simulink model "acdcmg_sim8_1_sm_grid_simulation"  (R2019b)
settings: Solver=ode8  StartTime=0.0  StopTime=0.5  FixedStep=4e-05  MaxStep=1e-2  RelTol=1e-3
PreLoadFcn:
  | Set_parameters_R2018
InitFcn:
  | Set_parameters_R2018
undefined symbols (not defined in the file or in its folder): D1, Delta, dis11, dis12, dis2, dis3, dis4, dis5, dis6, DiscIntNeverNeededParam, fn, Fnom, Ion, Lithium, max_min, P_Load_3, Pnom_T1, Pnom_T2, Pnom_T3, Ql_Load_3, R_Load_9, R_Load_DC, Rl, Rls, Ts, Ts_Control, Ts_Power, Ts_PV, V1_LL_T3, Vmin_mppt, VnInv, Vnom_DC, Vnom_Diesel, Vnom_prim, Vnom_sec, Vnom_ter_AC_DC, Xl, Xls
libraries: powerlib x136, powerlib_meascontrol x67, opal_lib x24, artemis x7, simulink x7, powerlib_extras x5, electricdrivelib x1, eeSinusoidalMeasurementV2 x1, re_lib x1
(part 4 of 4)

== system acdcmg_sim8_1_sm_grid_simulation/SM_Grid_Simulation/Bus_AC//DC3/Battery system/Ripple Calculations ==
  Signal : Inport
  Reset : Inport  Port=2
  0 : Constant  Value=2
  1 : Constant  Value=2
  Display10 : Display
  Display2 : Display
  Mean1 : powerlib_meascontrol/Measurements/Mean  Freq=10  Vinit=0  Ts=0
  MinMax Running Resettable : simulink/Math Operations/MinMax Running Resettable  Function=max  vinit=0.0
  MinMax Running Resettable1 : simulink/Math Operations/MinMax Running Resettable  Function=min  vinit=0.0
  Product : Product
  Product1 : Product
  Sum : Sum  Inputs=|+-
  Sum1 : Sum  Inputs=|-+
  Switch1 : Switch  Criteria=u2 > Threshold
  Switch2 : Switch  Criteria=u2 > Threshold
  Switch3 : Switch  Criteria=u2 > Threshold
  Ripple in Buck : Outport  VectorParamsAs1DForOutWhenUnconnected=off
  Ripple in Boost : Outport  Port=2  VectorParamsAs1DForOutWhenUnconnected=off
  wires:
  1/1 -> Product1/2
  [I_ref] -> Switch2/2, Switch3/2
  Product1/1 -> Switch3/3
  0/1 -> Product/2
  Switch2/1 -> Ripple in Buck/1
  Switch3/1 -> Ripple in Boost/1
  Product/1 -> Switch2/1
  Signal/1 -> Mean1/1, MinMax Running Resettable1/1, MinMax Running Resettable/1
  Switch1/1 -> Sum1/2, Sum/2
  MinMax Running Resettable/1 -> Sum/1, Display2/1
  MinMax Running Resettable1/1 -> Sum1/1, Display10/1
  Sum/1 -> Product/1
  Reset/1 -> Switch1/2, MinMax Running Resettable1/2, MinMax Running Resettable/2
  Sum1/1 -> Product1/1
  Mean1/1 -> Switch1/3

== system acdcmg_sim8_1_sm_grid_simulation/SM_Grid_Simulation/Bus_AC//DC3/PV system/Pmean ==
  Product : Product  RndMeth=Zero
  Scope : Scope  NumInputPorts=2
  W-kW : Gain  Gain=1/1000
  P : Outport  VectorParamsAs1DForOutWhenUnconnected=off
  V : Outport  Port=2  VectorParamsAs1DForOutWhenUnconnected=off
  wires:
  [Vdc_PV] -> Scope/1, Product/1, V/1
  Product/1 -> W-kW/1
  [Idc_PV] -> Scope/2, Product/2
  W-kW/1 -> P/1  "Pmean_PV (kW)"

== system acdcmg_sim8_1_sm_grid_simulation/SM_Grid_Simulation/Grid Bi-directional Converter 1.1 300 (DC) // 150 V (AC) P_nom 3kW2/Control of Inverter/Discrete PWM Generator1 ==
  note: Pierre Giroux, Gilbert Sybille
      | Power System Laboratory, IREQ
      | Hydro-Quebec
  note: PWM Generator
  Uref : Inport
  BL4 : Logic  Operator=NOT  Inputs=1
  BL5 : Logic  Operator=NOT  Inputs=1
  Constant : Constant  Value=Internal_Phase
  Constant1 : Constant  Value=Internal
  Data Type Conversion : DataTypeConversion  OutDataTypeStr=double  SaturateOnIntegerOverflow=on  RndMeth=Zero
  Data Type Conversion1 : DataTypeConversion  OutDataTypeStr=boolean  SaturateOnIntegerOverflow=on  RndMeth=Zero
  Data Type Conversion2 : DataTypeConversion  OutDataTypeStr=boolean  SaturateOnIntegerOverflow=on  RndMeth=Zero
  Gain : Gain  Gain=2*pi*Freq  SaturateOnIntegerOverflow=on  OutDataTypeStr=Inherit: Same as input  ParamDataTypeStr=Inherit: Same as input
  Gain2 : Gain  Gain=pi/180  SaturateOnIntegerOverflow=on  OutDataTypeStr=Inherit: Same as input  ParamDataTypeStr=Inherit: Same as input
  Gain3 : Gain  Gain=-1  SaturateOnIntegerOverflow=on  OutDataTypeStr=Inherit: Same as input  ParamDataTypeStr=Inherit: Same as input
  Mux : Mux  Inputs=2
  Mux1 : Mux  Inputs=2
  Mux2 : Mux  Inputs=2
  Product : Product  SaturateOnIntegerOverflow=on  InputSameDT=on  OutDataTypeStr=Inherit: Same as first input
  Relational Operator : RelationalOperator  RndMeth=Nearest  InputSameDT=on
  Relational Operator1 : RelationalOperator  RndMeth=Nearest  InputSameDT=on
  Select1A : Selector  InputPortWidth=Select1_PortWidth  IndexOptions=Index vector (dialog)  Indices=Select1_Elements  OutputSizes=1
  Select1B : Selector  InputPortWidth=Select1_PortWidth  IndexOptions=Index vector (dialog)  Indices=Select1_Elements  OutputSizes=1
  Select3 : Selector  InputPortWidth=Select3_PortWidth  IndexOptions=Index vector (dialog)  Indices=Select3_Elements  OutputSizes=1
  Sum : Sum  Inputs=+++  SaturateOnIntegerOverflow=on  InputSameDT=on  OutDataTypeStr=Inherit: Same as first input
  Switch : Switch  Criteria=u2 > Threshold
  Triangle : simulink/Sources/Repeating Sequence  rep_seq_t=[0 1/Fc/4 3/Fc/4 1/Fc]  rep_seq_y=[0 -1 1 0]
  Trigonometric Function : Trigonometry
  m3 : Constant  Value=Phase
  m4 : Constant  Value=mIndex
  t : DigitalClock  SampleTime=Ts
  Pulses : Outport  VectorParamsAs1DForOutWhenUnconnected=off
  wires:
  Mux2/1 -> Select3/1
  Select1B/1 -> Mux2/2
  Select1A/1 -> Mux2/1
  Mux1/1 -> Select1B/1
  Mux/1 -> Select1A/1
  BL5/1 -> Mux1/2
  BL4/1 -> Mux/2
  Gain3/1 -> Relational Operator1/1
  Triangle/1 -> Relational Operator1/2, Relational Operator/2
  Product/1 -> Switch/1
  Constant1/1 -> Switch/2
  Trigonometric Function/1 -> Product/2
  Sum/1 -> Trigonometric Function/1
  m4/1 -> Product/1
  Constant/1 -> Sum/3
  m3/1 -> Gain2/1
  Gain2/1 -> Sum/2
  Gain/1 -> Sum/1
  t/1 -> Gain/1
  Select3/1 -> Data Type Conversion/1
  Data Type Conversion/1 -> Pulses/1
  Relational Operator/1 -> Data Type Conversion1/1
  Data Type Conversion1/1 -> BL4/1, Mux/1
  Relational Operator1/1 -> Data Type Conversion2/1
  Data Type Conversion2/1 -> BL5/1, Mux1/1
  Switch/1 -> Relational Operator/1, Gain3/1
  Uref/1 -> Switch/3

== system acdcmg_sim8_1_sm_grid_simulation/SM_Grid_Simulation/Grid Bi-directional Converter 1.1 300 (DC) // 150 V (AC) P_nom 3kW2/Control of Inverter/MI Controller ==
  Vabc : Inport
  Demux : Demux  Commented=on  Outputs=3
  Demux1 : Demux  Outputs=3
  Mux : Mux  Inputs=3
  Mux1 : Mux  Inputs=3
  Mux2 : Mux  Inputs=3
  OP max / min : Subsystem
  Product : Product  RndMeth=Zero
  Product1 : Product  RndMeth=Zero
  Product2 : Product  RndMeth=Zero
  Subsystem : Subsystem
  Subsystem1 : Subsystem
  Terminator : Terminator
  Terminator1 : Terminator  Commented=on
  Terminator2 : Terminator  Commented=on
  Terminator3 : Terminator
  Terminator4 : Terminator  Commented=on
  Vab1 : powerlib_extras/Discrete Measurements/Discrete  RMS value  Commented=on  Freq=60  Mag_Init=0  Ts=20e-6
      settings: SourceProductBaseCode=PS
  Vab5 : powerlib_extras/Discrete Measurements/Discrete  RMS value  Commented=on  Freq=60  Mag_Init=0  Ts=20e-6
      settings: SourceProductBaseCode=PS
  Vab6 : powerlib_extras/Discrete Measurements/Discrete  RMS value  Commented=on  Freq=60  Mag_Init=0  Ts=20e-6
      settings: SourceProductBaseCode=PS
  Vabc_inv : Outport  VectorParamsAs1DForOutWhenUnconnected=off
  u / m : Outport  Port=2  VectorParamsAs1DForOutWhenUnconnected=off
  wires:
  Product/1 -> Mux2/1
  Product1/1 -> Mux2/2
  Product2/1 -> Mux2/3
  Mux1/1 -> u / m/1
  Vabc/1 -> Demux/1
  Demux/1 -> Vab6/1
  Demux/2 -> Vab5/1
  Demux/3 -> Vab1/1
  Demux1/1 -> Product/1, Mux1/1
  Demux1/2 -> Product1/1, Mux1/2
  Demux1/3 -> Product2/1, Mux1/3
  Subsystem/1(Va) -> Product/2
  Subsystem/2(Vb) -> Product1/2
  Subsystem/3(Vc) -> Product2/2
  Mux2/1 -> Vabc_inv/1
  Vab6/1 -> Terminator2/1
  Subsystem1/3(wt) -> Terminator/1
  Subsystem1/1(Frec) -> Terminator3/1
  Subsystem1/2(sin_cos) -> Subsystem/1(sin_cos)
  Mux/1 -> Demux1/1
  OP max / min/1(ctrl) -> Mux/3, Mux/1, Mux/2
  Vab5/1 -> Terminator1/1
  Vab1/1 -> Terminator4/1

== system acdcmg_sim8_1_sm_grid_simulation/SM_Grid_Simulation/Inverter 300 (DC) // 150 V (AC) P_nom 10 kW4/Control of Inverter/Positive-Sequence Active & Reactive Power1 ==
  note: Discrete 3-phase Positive-Sequence Active & Reactive Power
  note: Pierre Giroux, Gilbert Sybille
      | Power System Simulation Laboratory
      | IREQ, Hydro-Quebc
  Vabc : Inport  PortDimensions=3
  Iabc : Inport  Port=2  PortDimensions=3
  Deg->Rad : Gain  Gain=pi/180  SaturateOnIntegerOverflow=on  OutDataTypeStr=Inherit: Same as input  ParamDataTypeStr=Inherit: Same as input
  Discrete 3-phase Positive-Sequence Fundamental Value (I) : powerlib_extras/Discrete Measurements/Discrete 3-phase Positive-Sequence Fundamental Value  Freq=Freq  Par_Init=Par_Iinit  Ts=Ts
      settings: SourceProductBaseCode=PS
  Discrete 3-phase Positive-Sequence Fundamental Value (V) : powerlib_extras/Discrete Measurements/Discrete 3-phase Positive-Sequence Fundamental Value  Freq=Freq  Par_Init=Par_Vinit  Ts=Ts
      settings: SourceProductBaseCode=PS
  Gain1 : Gain  Gain=3/2  SaturateOnIntegerOverflow=on  OutDataTypeStr=Inherit: Same as input  ParamDataTypeStr=Inherit: Same as input
  Mag->RMS : Gain  Gain=1/sqrt(2)
  Mux1 : Mux  Inputs=2
  Mux2 : Mux  Inputs=2
  Mux3 : Mux  Inputs=2
  Product : Product  SaturateOnIntegerOverflow=on  InputSameDT=on  OutDataTypeStr=Inherit: Same as first input
  Product1 : Product  SaturateOnIntegerOverflow=on  InputSameDT=on  OutDataTypeStr=Inherit: Same as first input
  Product2 : Product  SaturateOnIntegerOverflow=on  InputSameDT=on  OutDataTypeStr=Inherit: Same as first input
  Sum : Sum  Inputs=+-  SaturateOnIntegerOverflow=on  InputSameDT=on  OutDataTypeStr=Inherit: Same as first input
  Trigonometric Function : Trigonometry
  Trigonometric Function1 : Trigonometry  Operator=cos
  W->kW Var->kvar : Gain  Gain=1/1000
  RMS_V_I : Outport
  P_Q(kW) : Outport  Port=2
  Phase_V_I : Outport  Port=3
  PF : Outport  Port=4
  wires:
  Vabc/1 -> Discrete 3-phase Positive-Sequence Fundamental Value (V)/1
  Iabc/1 -> Discrete 3-phase Positive-Sequence Fundamental Value (I)/1
  Discrete 3-phase Positive-Sequence Fundamental Value (V)/2 -> Sum/1, Mux1/1
  Discrete 3-phase Positive-Sequence Fundamental Value (I)/2 -> Sum/2, Mux1/2
  Sum/1 -> Deg->Rad/1
  Deg->Rad/1 -> Trigonometric Function1/1, Trigonometric Function/1
  Trigonometric Function1/1 -> PF/1, Product/2
  Trigonometric Function/1 -> Product1/1
  Mux2/1 -> Gain1/1
  Product/1 -> Mux2/1
  Product1/1 -> Mux2/2
  Product2/1 -> Product/1, Product1/2
  Discrete 3-phase Positive-Sequence Fundamental Value (V)/1 -> Mux3/1, Product2/1
  Discrete 3-phase Positive-Sequence Fundamental Value (I)/1 -> Mux3/2, Product2/2
  Mux1/1 -> Phase_V_I/1
  Mux3/1 -> Mag->RMS/1
  Mag->RMS/1 -> RMS_V_I/1
  Gain1/1 -> W->kW Var->kvar/1
  W->kW Var->kvar/1 -> P_Q(kW)/1

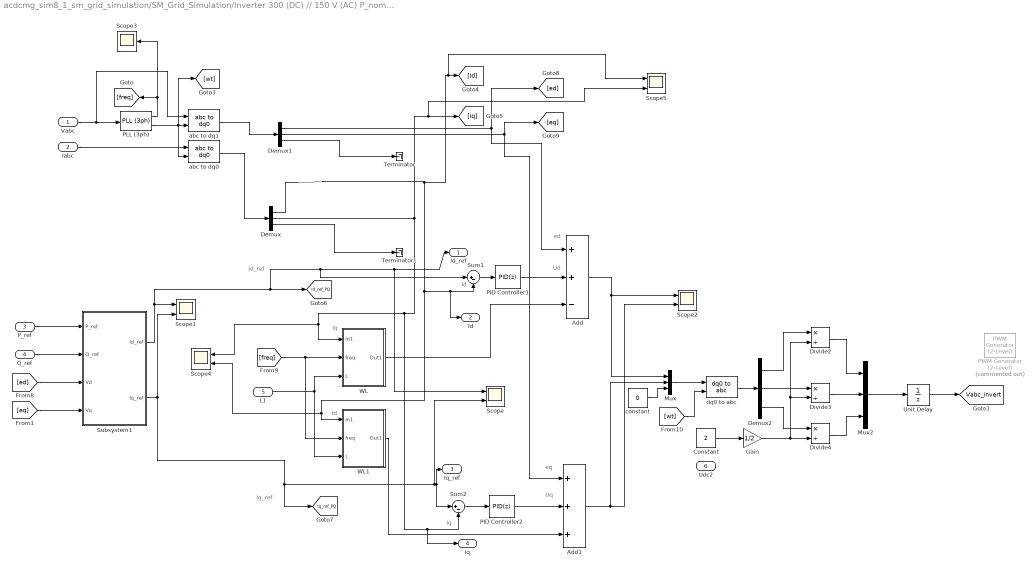
== system acdcmg_sim8_1_sm_grid_simulation/SM_Grid_Simulation/Inverter 300 (DC) // 150 V (AC) P_nom 10 kW4/Control of Inverter/Subsystem2 ==
  note: Iq_ref
  note: Id
  note: Id_ref
  note: Ud
  note: Uq
  note: eq
  note: ed
  note: Iq
  note: Id
  note: Iq
  Vabc : Inport
  Iabc : Inport  Port=2
  P_ref : Inport  Port=3
  Q_ref : Inport  Port=4
  L1 : Inport  Port=5
  Udc2 : Inport  Port=6
  Add : Sum  Inputs=++-
  Add1 : Sum  Inputs=+++
  Constant : Constant  Value=2
  Demux : Demux  Outputs=3
  Demux1 : Demux  Outputs=3
  Demux2 : Demux  Outputs=3
  Divide2 : Product  Inputs=*/
  Divide3 : Product  Inputs=*/
  Divide4 : Product  Inputs=*/
  Gain : Gain  Gain=1/2
  Mux : Mux  Inputs=3
  Mux2 : Mux  Inputs=3
  PID Controller1 : simulink/Continuous/PID Controller  Controller=PID  Form=Parallel  TimeDomain=Discrete-time  SampleTime=Ts_Control  IntegratorMethod=Forward Euler  FilterMethod=Forward Euler  ControllerParametersSource=internal  P=Kp  I=Ki  D=Kd  UseFilter=on  N=100  TunerSelectOption=Transfer Function Based (PID Tuner App)  InitialConditionSource=internal  InitialConditionForIntegrator=0  InitialConditionForFilter=0  DifferentiatorICPrevScaledInput=0  ExternalReset=none  TrackingMode=off  Kt=1  LimitOutput=off  UpperSaturationLimit=inf  LowerSaturationLimit=-inf  LinearizeAsGain=on  AntiWindupMode=none  Kb=1  POutMin=[]  POutMax=[]  IOutMin=[]  IOutMax=[]  DOutMin=[]  DOutMax=[]  NOutMin=[]  NOutMax=[]  SumOutMin=[]  SumOutMax=[]  SaturationOutMin=[]  SaturationOutMax=[]  PParamMin=[]  PParamMax=[]  IParamMin=[]  IParamMax=[]  DParamMin=[]  DParamMax=[]  NParamMin=[]  NParamMax=[]  KbParamMin=[]  KbParamMax=[]  KtParamMin=[]  KtParamMax=[]  KbOutMin=[]  KbOutMax=[]  KtOutMin=[]  KtOutMax=[]  IntegratorOutMin=[]  IntegratorOutMax=[]  FilterOutMin=[]  FilterOutMax=[]  SumI1OutMin=[]  SumI1OutMax=[]  SumI2OutMin=[]  SumI2OutMax=[]  SumI3OutMin=[]  SumI3OutMax=[]  SumI4OutMin=[]  SumI4OutMax=[]  SumDOutMin=[]  SumDOutMax=[]  DifferentiatorOutMin=[]  DifferentiatorOutMax=[]  FilterDiffOutCoefMin=[]  FilterDiffOutCoefMax=[]  ReciprocalOutMin=[]  ReciprocalOutMax=[]  SumDenOutMin=[]  SumDenOutMax=[]  SumNumOutMin=[]  SumNumOutMax=[]  DivideOutMin=[]  DivideOutMax=[]  IntegratorContinuousStateAttributes=''  IntegratorStateMustResolveToSignalObject=off  IntegratorRTWStateStorageClass=Auto  FilterContinuousStateAttributes=''  FilterStateMustResolveToSignalObject=off  FilterRTWStateStorageClass=Auto  ParallelPVariant=InternalParameters  IdealPVariant=Disabled  IVariant=InternalParameters  DVariant=InternalParameters  IntegratorVariant=Discrete  SatVariant=Disabled  AWVariant=Passthrough  PCopyVariant=Disabled  TRVariant=Disabled  FdbkBlocksVariant=Forward  IdealPFdbkVariant=Disabled  SatFdbkVariant=Disabled  DerivativeFilterVariant=ForwardEulerFilter  NVariant=InternalParameters  NCopyVariant=Disabled  FilterICVariant=InternalICsFilter  IntegratorICVariant=InternalICs  ExternalResetVariant=Disabled  TRSumVariant=Passthrough  SumFdbkVariant=Disabled  SumVariant=Sum_PID
  PID Controller2 : simulink/Continuous/PID Controller  Controller=PID  Form=Parallel  TimeDomain=Discrete-time  SampleTime=Ts_Control  IntegratorMethod=Forward Euler  FilterMethod=Forward Euler  ControllerParametersSource=internal  P=Kp  I=Ki  D=Kd  UseFilter=on  N=100  TunerSelectOption=Transfer Function Based (PID Tuner App)  InitialConditionSource=internal  InitialConditionForIntegrator=0  InitialConditionForFilter=0  DifferentiatorICPrevScaledInput=0  ExternalReset=none  TrackingMode=off  Kt=1  LimitOutput=off  UpperSaturationLimit=inf  LowerSaturationLimit=-inf  LinearizeAsGain=on  AntiWindupMode=none  Kb=1  POutMin=[]  POutMax=[]  IOutMin=[]  IOutMax=[]  DOutMin=[]  DOutMax=[]  NOutMin=[]  NOutMax=[]  SumOutMin=[]  SumOutMax=[]  SaturationOutMin=[]  SaturationOutMax=[]  PParamMin=[]  PParamMax=[]  IParamMin=[]  IParamMax=[]  DParamMin=[]  DParamMax=[]  NParamMin=[]  NParamMax=[]  KbParamMin=[]  KbParamMax=[]  KtParamMin=[]  KtParamMax=[]  KbOutMin=[]  KbOutMax=[]  KtOutMin=[]  KtOutMax=[]  IntegratorOutMin=[]  IntegratorOutMax=[]  FilterOutMin=[]  FilterOutMax=[]  SumI1OutMin=[]  SumI1OutMax=[]  SumI2OutMin=[]  SumI2OutMax=[]  SumI3OutMin=[]  SumI3OutMax=[]  SumI4OutMin=[]  SumI4OutMax=[]  SumDOutMin=[]  SumDOutMax=[]  DifferentiatorOutMin=[]  DifferentiatorOutMax=[]  FilterDiffOutCoefMin=[]  FilterDiffOutCoefMax=[]  ReciprocalOutMin=[]  ReciprocalOutMax=[]  SumDenOutMin=[]  SumDenOutMax=[]  SumNumOutMin=[]  SumNumOutMax=[]  DivideOutMin=[]  DivideOutMax=[]  IntegratorContinuousStateAttributes=''  IntegratorStateMustResolveToSignalObject=off  IntegratorRTWStateStorageClass=Auto  FilterContinuousStateAttributes=''  FilterStateMustResolveToSignalObject=off  FilterRTWStateStorageClass=Auto  ParallelPVariant=InternalParameters  IdealPVariant=Disabled  IVariant=InternalParameters  DVariant=InternalParameters  IntegratorVariant=Discrete  SatVariant=Disabled  AWVariant=Passthrough  PCopyVariant=Disabled  TRVariant=Disabled  FdbkBlocksVariant=Forward  IdealPFdbkVariant=Disabled  SatFdbkVariant=Disabled  DerivativeFilterVariant=ForwardEulerFilter  NVariant=InternalParameters  NCopyVariant=Disabled  FilterICVariant=InternalICsFilter  IntegratorICVariant=InternalICs  ExternalResetVariant=Disabled  TRSumVariant=Passthrough  SumFdbkVariant=Disabled  SumVariant=Sum_PID
  PLL (3ph) : powerlib_meascontrol/PLL/PLL (3ph)  Fmin=59.5  Par_Init=[0, 60]  ParK=[180, 3200, 1]  TcD=2.5e-4  MaxRateChangeFreq=12  FilterCutOffFreq=25  Ts=Ts_Control  AGC=on
  PWM Generator (2-Level) : powerlib_meascontrol/Pulse & Signal Generators/PWM Generator (2-Level)  Commented=on  ModulatorType=Three-phase bridge (6 pulses)  ModulatorMode=Unsynchronized  Fc=15000  Pc=90  nF=27  MinMax="[ -1  1 ]"  SamplingTechnique=Natural  ModulatingSignals=off  m=0.8  Freq=60  Phase=0  Ts=Ts_Power  ShowCarrierOutport=off
  Scope{,1..2,4..5} (5 alike) : Scope  NumInputPorts=2
  Scope3 : Scope
  Subsystem1 : Subsystem
  Sum1 : Sum  Inputs=|+-
  Sum2 : Sum  Inputs=|+-
  Terminator : Terminator
  Terminator1 : Terminator
  Unit Delay : UnitDelay  SampleTime=-1  HasFrameUpgradeWarning=on
  WL : Subsystem
  WL1 : Subsystem
  abc to dq0 : powerlib_meascontrol/Transformations/abc to dq0  Alignment=90 degrees behind phase A axis
  abc to dq1 : powerlib_meascontrol/Transformations/abc to dq0  Alignment=90 degrees behind phase A axis
  constant : Constant  Value=0
  dq0 to abc : powerlib_meascontrol/Transformations/dq0 to abc  Alignment=90 degrees behind phase A axis
  Id_ref : Outport
  Id : Outport  Port=2
  Iq_ref : Outport  Port=3
  Iq : Outport  Port=4
  tag scope: Id_ref_PQ=global, Iq_ref_PQ=global, Vabc_invert=global
  wires:
  abc to dq1/1 -> Demux1/1
  Sum1/1 -> PID Controller1/1
  Iabc/1 -> abc to dq0/1
  Vabc/1 -> abc to dq1/1, PLL (3ph)/1
  PLL (3ph)/2 -> [wt], abc to dq1/2, abc to dq0/2
  Demux1/1 -> Add/1, [ed]
  L1/1 -> WL/3(L), WL1/3(L)
  WL/1(Out1) -> Add/3
  [freq] -> WL1/2(freq), WL/2(freq)
  PLL (3ph)/1 -> Scope3/1, [freq]
  Demux2/1 -> Divide2/1
  Add/1 -> Mux/1, Scope2/1
  PID Controller2/1 -> Add1/2
  Sum2/1 -> PID Controller2/1
  Demux2/2 -> Divide3/1
  WL1/1(Out1) -> Add1/3
  Demux1/2 -> Add1/1, [eq]
  Add1/1 -> Mux/2, Scope2/2
  Gain/1 -> Divide3/2, Divide2/2, Divide4/2
  Divide4/1 -> Mux2/3
  Divide2/1 -> Mux2/1
  Mux/1 -> dq0 to abc/1
  Demux2/3 -> Divide4/1
  Divide3/1 -> Mux2/2
  dq0 to abc/1 -> Demux2/1
  PID Controller1/1 -> Add/2
  [wt] -> dq0 to abc/2
  Demux1/3 -> Terminator/1
  Demux/3 -> Terminator1/1
  constant/1 -> Mux/3
  P_ref/1 -> Subsystem1/1(P_ref)
  Q_ref/1 -> Subsystem1/2(Q_ref)
  [ed] -> Subsystem1/3(Vd)
  [eq] -> Subsystem1/4(Vq)
  Subsystem1/2(Iq_ref) -> Scope1/2, [Iq_ref_PQ], Scope/2, Iq_ref/1, Sum2/1
  Subsystem1/1(Id_ref) -> Sum1/1, Scope/1, Id_ref/1, [Id_ref_PQ], Scope1/1
  Demux/1 -> Scope4/2, WL1/1(In1), Id/1, Sum1/2, Scope5/1, [Id]
  Demux/2 -> Scope5/2, [Iq], Scope4/1, WL/1(In1), Iq/1, Sum2/2
  abc to dq0/1 -> Demux/1
  Mux2/1 -> Unit Delay/1
  Unit Delay/1 -> [Vabc_invert]
  Constant/1 -> Gain/1

== system acdcmg_sim8_1_sm_grid_simulation/SM_Grid_Simulation/OpComm1/busStruct/Sub1 ==
  in : Inport
  out : Outport
  wires:
  in/1 -> out/1  "signal1"

== system acdcmg_sim8_1_sm_grid_simulation/SM_Grid_Simulation/OpComm1/busStruct/Sub2 ==
  in : Inport
  out : Outport
  wires:
  in/1 -> out/1  "signal1"

== system acdcmg_sim8_1_sm_grid_simulation/SM_Grid_Simulation/OpComm1/busStruct/Sub3 ==
  in : Inport
  out : Outport
  wires:
  in/1 -> out/1  "signal1"

== system acdcmg_sim8_1_sm_grid_simulation/SM_Grid_Simulation/OpComm1/busStruct/Sub4 ==
  in : Inport
  out : Outport
  wires:
  in/1 -> out/1  "signal1"

== system acdcmg_sim8_1_sm_grid_simulation/SM_Grid_Simulation/OpComm1/busStruct/Sub5 ==
  in : Inport
  out : Outport
  wires:
  in/1 -> out/1  "signal1"

== system acdcmg_sim8_1_sm_grid_simulation/SM_Grid_Simulation/OpComm1/busStruct/Sub6 ==
  in : Inport
  out : Outport
  wires:
  in/1 -> out/1  "signal1"

== system acdcmg_sim8_1_sm_grid_simulation/SM_Grid_Simulation/OpComm1/busStruct/Sub7 ==
  in : Inport
  out : Outport
  wires:
  in/1 -> out/1  "signal1"

== system acdcmg_sim8_1_sm_grid_simulation/SM_Grid_Simulation/OpComm1/busStruct/Sub8 ==
  in : Inport
  out : Outport
  wires:
  in/1 -> out/1  "signal1"

== system acdcmg_sim8_1_sm_grid_simulation/SM_Grid_Simulation/Grid Bi-directional Converter 1.1 300 (DC) // 150 V (AC) P_nom 3kW2/Control of Inverter/MI Controller/OP max // min ==
  note: DC to AC
  note: AC to DC
  Constant2 : Constant  Value=max_min
  OP_max1 : Constant  Value=1.2
  OP_min1 : Constant
  Switch2 : Switch  Criteria=u2 > Threshold
  ctrl : Outport  VectorParamsAs1DForOutWhenUnconnected=off
  wires:
  OP_max1/1 -> Switch2/1
  OP_min1/1 -> Switch2/3
  Constant2/1 -> Switch2/2
  Switch2/1 -> ctrl/1

== system acdcmg_sim8_1_sm_grid_simulation/SM_Grid_Simulation/Grid Bi-directional Converter 1.1 300 (DC) // 150 V (AC) P_nom 3kW2/Control of Inverter/MI Controller/Subsystem ==
  sin_cos : Inport  PortDimensions=2
  Demux : Demux  Outputs=2
  Fcn2 : Fcn  Expr=1*u[1]
  Fcn4 : Fcn  Expr=1*u[3]
  Fcn5 : Fcn  Expr=1*u[5]
  K1 : Constant  Value=0.5
  K2 : Constant  Value=sqrt(3)/2
  Mux2 : Mux  Inputs=6
  Product{,1..3} (4 alike) : Product  SaturateOnIntegerOverflow=on  InputSameDT=on  OutDataTypeStr=Inherit: Same as first input
  Sum : Sum  Inputs=--  SaturateOnIntegerOverflow=on  InputSameDT=on  OutDataTypeStr=Inherit: Same as first input
  Sum1 : Sum  Inputs=-+  SaturateOnIntegerOverflow=on  InputSameDT=on  OutDataTypeStr=Inherit: Same as first input
  Sum2 : Sum  Inputs=--  SaturateOnIntegerOverflow=on  InputSameDT=on  OutDataTypeStr=Inherit: Same as first input
  Sum3 : Sum  Inputs=--  SaturateOnIntegerOverflow=on  InputSameDT=on  OutDataTypeStr=Inherit: Same as first input
  Va : Outport  VectorParamsAs1DForOutWhenUnconnected=off
  Vb : Outport  Port=2  VectorParamsAs1DForOutWhenUnconnected=off
  Vc : Outport  Port=3  VectorParamsAs1DForOutWhenUnconnected=off
  wires:
  sin_cos/1 -> Demux/1
  Demux/1 -> Product/1, Product2/1, Sum2/2, Mux2/1  "sin(wt)"
  Product/1 -> Sum/1
  Product1/1 -> Sum/2
  Product3/1 -> Sum1/1
  Product2/1 -> Sum1/2
  Sum3/1 -> Mux2/6  "cos(wt+2pi/3)"
  Sum2/1 -> Mux2/5  "sin(wt+2pi/3)"
  K1/1 -> Product/2, Product3/2
  K2/1 -> Product1/2, Product2/2
  Sum/1 -> Mux2/3, Sum2/1  "sin(wt-2pi/3)"
  Sum1/1 -> Mux2/4, Sum3/1  "cos(wt-2pi/3)"
  Demux/2 -> Sum3/2, Product3/1, Product1/1, Mux2/2  "cos(wt)"
  Mux2/1 -> Fcn2/1, Fcn4/1, Fcn5/1
  Fcn2/1 -> Va/1
  Fcn4/1 -> Vb/1
  Fcn5/1 -> Vc/1

== system acdcmg_sim8_1_sm_grid_simulation/SM_Grid_Simulation/Grid Bi-directional Converter 1.1 300 (DC) // 150 V (AC) P_nom 3kW2/Control of Inverter/MI Controller/Subsystem1 ==
  note: AC to DC
  note: DC to AC
  Constant1 : Constant  Value=max_min
  Constant2 : Constant  Value=2*pi
  Deg->Rad : Gain  Gain=pi/180  SaturateOnIntegerOverflow=on  OutDataTypeStr=Inherit: Same as input  ParamDataTypeStr=Inherit: Same as input
  Freq1 : Constant  Value=Fnom
  Freq2 : Constant  Value=2*pi
  Math Function : Math  Operator=mod  SaturateOnIntegerOverflow=on
  Mux5 : Mux  Inputs=2
  OP_max1 : Constant  Value=0
  OP_min1 : Constant  Value=228
  Product7 : Product  Inputs=***  SaturateOnIntegerOverflow=on  InputSameDT=on  OutDataTypeStr=Inherit: Same as first input
  Sum : Sum  SaturateOnIntegerOverflow=on  InputSameDT=on  OutDataTypeStr=Inherit: Same as first input
  Switch2 : Switch  Criteria=u2 > Threshold
  Trigonometric Function : Trigonometry
  Trigonometric Function1 : Trigonometry  Operator=cos
  t : DigitalClock  SampleTime=Ts
  Frec : Outport  VectorParamsAs1DForOutWhenUnconnected=off
  sin_cos : Outport  Port=2  VectorParamsAs1DForOutWhenUnconnected=off
  wt : Outport  Port=3  VectorParamsAs1DForOutWhenUnconnected=off
  wires:
  Switch2/1 -> Deg->Rad/1
  Deg->Rad/1 -> Sum/2
  Freq1/1 -> Frec/1, Product7/1
  Trigonometric Function/1 -> Mux5/1
  Sum/1 -> Math Function/1
  Trigonometric Function1/1 -> Mux5/2
  Product7/1 -> Sum/1
  Freq2/1 -> Product7/3
  Constant2/1 -> Math Function/2
  t/1 -> Product7/2
  Math Function/1 -> wt/1, Trigonometric Function1/1, Trigonometric Function/1
  Mux5/1 -> sin_cos/1
  Constant1/1 -> Switch2/2
  OP_max1/1 -> Switch2/1
  OP_min1/1 -> Switch2/3

== system acdcmg_sim8_1_sm_grid_simulation/SM_Grid_Simulation/Inverter 300 (DC) // 150 V (AC) P_nom 10 kW4/Control of Inverter/Subsystem2/Subsystem1 ==
  note: Iq* = 2/3*( P*Vq - Q*Vd ) / ( Vd^2 + Vq^2 )
  note: Reference computation:
  note: Id* = 2/3* ( P*Vd + Q*Vq ) / ( Vd^2 + Vq^2 )
  P_ref : Inport  PortDimensions=1
  Q_ref : Inport  Port=2  PortDimensions=1
  Vd : Inport  Port=3  PortDimensions=1
  Vq : Inport  Port=4  PortDimensions=1
  Constant1 : Constant  Commented=on  Value=0
  Demux3 : Demux  Outputs=2
  Fcn3 : Fcn  Expr=u(1)*u(1)+u(2)*u(2)
  Gain : Gain  Gain=2/3
  Mux1 : Mux  Inputs=2
  Mux3 : Mux  Inputs=2
  Product{2..5} (4 alike) : Product  SaturateOnIntegerOverflow=on  InputSameDT=on  OutDataTypeStr=Inherit: Same as first input
  Product6 : Product  Inputs=*/  SaturateOnIntegerOverflow=on  InputSameDT=on  OutDataTypeStr=Inherit: Same as first input
  Scope3 : Scope  NumInputPorts=2
  Sum : Sum  SaturateOnIntegerOverflow=on  InputSameDT=on  OutDataTypeStr=Inherit: Same as first input
  Sum1 : Sum  Inputs=+-  SaturateOnIntegerOverflow=on  InputSameDT=on  OutDataTypeStr=Inherit: Same as first input
  Terminator : Terminator  Commented=on
  Id_ref : Outport
  Iq_ref : Outport  Port=2
  wires:
  Vq/1 -> Mux1/2, Product4/2, Product3/1
  Demux3/1 -> Scope3/1, Id_ref/1
  Mux1/1 -> Fcn3/1
  Product3/1 -> Sum/2
  Mux3/1 -> Gain/1
  Vd/1 -> Mux1/1, Product5/2, Product2/1
  Product4/1 -> Sum1/1
  Product6/1 -> Demux3/1
  Fcn3/1 -> Product6/2
  Demux3/2 -> Scope3/2, Iq_ref/1
  P_ref/1 -> Product2/2, Product4/1
  Gain/1 -> Product6/1
  Product2/1 -> Sum/1
  Q_ref/1 -> Product5/1, Product3/2
  Sum1/1 -> Mux3/2
  Product5/1 -> Sum1/2
  Sum/1 -> Mux3/1

== system acdcmg_sim8_1_sm_grid_simulation/SM_Grid_Simulation/Inverter 300 (DC) // 150 V (AC) P_nom 10 kW4/Control of Inverter/Subsystem2/WL ==
  In1 : Inport
  freq : Inport  Port=2
  L : Inport  Port=3
  2pai : Constant  Value=2*pi
  Product : Product  Inputs=**
  Product1 : Product  Inputs=***
  Out1 : Outport
  wires:
  2pai/1 -> Product/2
  L/1 -> Product1/3
  freq/1 -> Product/1
  Product1/1 -> Out1/1
  Product/1 -> Product1/2
  In1/1 -> Product1/1

== system acdcmg_sim8_1_sm_grid_simulation/SM_Grid_Simulation/Inverter 300 (DC) // 150 V (AC) P_nom 10 kW4/Control of Inverter/Subsystem2/WL1 ==
  In1 : Inport
  freq : Inport  Port=2
  L : Inport  Port=3
  2pai : Constant  Value=2*pi
  Product : Product
  Product1 : Product  Inputs=3
  Out1 : Outport
  wires:
  2pai/1 -> Product/2
  L/1 -> Product1/3
  freq/1 -> Product/1
  Product1/1 -> Out1/1
  Product/1 -> Product1/2
  In1/1 -> Product1/1
